simulink model "FeedbackLin"  (R2016a)
settings: Solver=ode45  StartTime=0.0  StopTime=2*Tpasso  FixedStep=1e-4  RelTol=1e-5
values from neighbouring files (symbols this model uses):
  Bm = 1e-4    (= 0.0001)    [runTests.m]
  cm = [c1; c2; c3; c4; c5]    [runTests.m]
  Cphi = 1    [runTests.m]
  cr = [c1; c2; c3; c4; c5]    [runTests.m]
  dQ0 = [dQ10; dQ20; dQ30; dQ40; dQ50]    [runNoErrorNoNoiseNoIncNoFext.m]    (also in runTests.m = zeros(5,1))
  gait = 1    [runTests.m]
  gm = g    (= 9.81)    [runTests.m]
  gr = g    (= 9.81)    [runTests.m]
  Im = [I1; I2; I3; I4; I5]    [runTests.m]
  Ir = [I1; I2; I3; I4; I5]    [runTests.m]
  Jm = 5e-3    (= 0.005)    [runTests.m]
  Kt = 0.1    [runTests.m]
  La = 1e-3    (= 0.001)    [runTests.m]
  LambdaFL = [150; 150; 150; 150]    [runTests.m]
  lm = [l1; l2; l3; l4; l5]    [runTests.m]
  lr = [l1; l2; l3; l4; l5]    [runTests.m]
  mInc = tan(Inc*pi/180)    [runTests.m]
  mm = [m1; m2; m3; m4; m5]    [runTests.m]
  mr = [m1; m2; m3; m4; m5]    [runTests.m]
  pertAmp = 0    [runTests.m]
  pertDur = 0    [runTests.m]
  pertStep = 0    [runTests.m]
  Q0 = [Q10; Q20; Q30; Q40; Q50]    [runNoErrorNoNoiseNoIncNoFext.m]    (also in runTests.m = [pi/2 - pi/10; pi/5; 2*pi-pi/10; pi+pi/10; -pi/4.5])
  Ra = 1    [runTests.m]
  Tpasso = 0.35    [runTests.m]
  TsC = 0.003    [runTests.m]
  TsPID = 1/1000    (= 0.001)    [runTests.m]
  useNoise = false    [runTests.m]
undefined symbols (not defined in the file or in its folder): curStep, Rp1, Rp2
libraries: simulink x8, commrandsrc3 x2
(part 1 of 3)
settings Model: Creator=PPA  LastModifiedBy=Barth

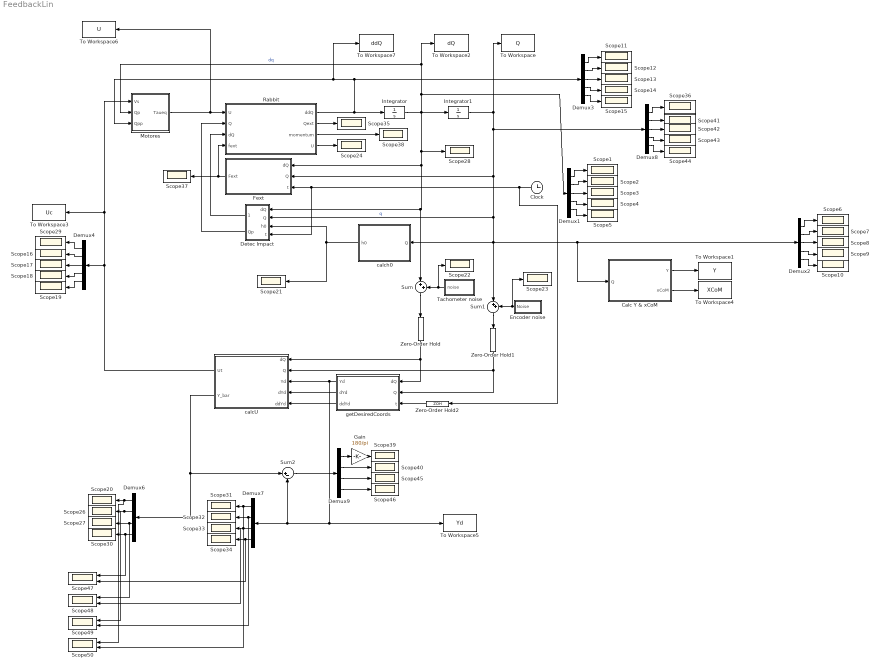
== system FeedbackLin ==
  Calc Y & xCoM : MATLAB Function  TreatAsAtomicUnit=on  SystemSampleTime=TsC
  Clock : Clock
  Demux{1..4,8} (5 alike) : Demux  Outputs=5
  Demux6 : Demux
  Demux7 : Demux
  Demux9 : Demux
  Detec Impact : Subsystem
  Encoder noise : Subsystem
  Fext : MATLAB Function  TreatAsAtomicUnit=on
  Gain : Gain  Gain=180/pi
  Integrator : Integrator  InitialCondition=dQ0
  Integrator1 : Integrator  InitialCondition=Q0
  Motores : Subsystem
  Rabbit : MATLAB Function  TreatAsAtomicUnit=on
  Scope{1..24,26..46} (45 alike) : Scope
  Scope{47..50} (4 alike) : Scope  NumInputPorts=2
  Sum : Sum  Inputs=|++
  Sum1 : Sum  Inputs=|++
  Sum2 : Sum  Inputs=|+-
  Tachometer noise : Subsystem
  To Workspace : ToWorkspace  VariableName=Q  SaveFormat=Structure With Time  SampleTime=-1
  To Workspace1 : ToWorkspace  VariableName=Y  SaveFormat=Structure With Time  SampleTime=-1
  To Workspace2 : ToWorkspace  VariableName=dQ  SaveFormat=Structure With Time  SampleTime=-1
  To Workspace3 : ToWorkspace  VariableName=Uc  SaveFormat=Structure With Time  SampleTime=-1
  To Workspace4 : ToWorkspace  VariableName=XCoM  SaveFormat=Structure With Time  SampleTime=-1
  To Workspace5 : ToWorkspace  VariableName=Yd  SaveFormat=Structure With Time  SampleTime=-1
  To Workspace6 : ToWorkspace  VariableName=U  SaveFormat=Structure With Time  SampleTime=-1
  To Workspace7 : ToWorkspace  VariableName=ddQ  SaveFormat=Structure With Time  SampleTime=-1
  Zero-Order Hold : ZeroOrderHold  SampleTime=TsC
  Zero-Order Hold1 : ZeroOrderHold  SampleTime=TsC
  Zero-Order Hold2 : ZeroOrderHold  SampleTime=TsC
  calcU : MATLAB Function  TreatAsAtomicUnit=on  SystemSampleTime=TsC
  calch0 : MATLAB Function  TreatAsAtomicUnit=on
  getDesiredCoords : Subsystem
  wires:
  Demux3/1 -> Scope11/1
  Demux3/2 -> Scope12/1
  Demux3/3 -> Scope13/1
  Demux3/4 -> Scope14/1
  Demux3/5 -> Scope15/1
  Integrator/1 -> Motores/2(Qp), To Workspace2/1, Demux1/1, Fext/1(dQ), Detec Impact/1(dQ), Sum/1, Scope28/1, Integrator1/1  "dq"
  Integrator1/1 -> Fext/2(Q), Detec Impact/2(Q), Calc Y & xCoM/1(Q), Demux2/1, Sum1/1, calch0/1(Q), Demux8/1, To Workspace/1  "q"
  Demux1/1 -> Scope1/1
  Demux1/2 -> Scope2/1
  Demux1/3 -> Scope3/1
  Demux1/4 -> Scope4/1
  Demux1/5 -> Scope5/1
  Demux2/1 -> Scope6/1
  Demux2/2 -> Scope7/1
  Demux2/3 -> Scope8/1
  Demux2/4 -> Scope9/1
  Demux2/5 -> Scope10/1
  Fext/1(Fext) -> Rabbit/4(fext), Scope37/1
  Clock/1 -> Zero-Order Hold2/1, Fext/3(t), Detec Impact/4(t)
  Demux4/3 -> Scope17/1
  Demux4/2 -> Scope16/1
  Demux4/1 -> Scope29/1
  Demux4/4 -> Scope18/1
  Demux4/5 -> Scope19/1
  Sum/1 -> Zero-Order Hold/1
  Sum1/1 -> Zero-Order Hold1/1
  Rabbit/3(momentum) -> Scope38/1
  Tachometer noise/1(noise) -> Sum/2, Scope22/1
  Detec Impact/1(dQp) -> Rabbit/3(dQ)
  Detec Impact/2(Qp) -> Rabbit/2(Q)
  calch0/1(h0) -> Scope21/1, Detec Impact/3(h0)
  Rabbit/2(Qext) -> Scope35/1
  Rabbit/1(ddQ) -> Demux3/1, To Workspace7/1, Motores/3(Qpp), Integrator/1
  Demux8/1 -> Scope36/1
  Demux8/2 -> Scope41/1
  Demux8/3 -> Scope42/1
  Demux8/4 -> Scope43/1
  Demux8/5 -> Scope44/1
  getDesiredCoords/3(ddYd) -> calcU/5(ddYd)
  getDesiredCoords/2(dYd) -> calcU/4(dYd)
  getDesiredCoords/1(Yd) -> calcU/3(Yd), To Workspace5/1, Sum2/2, Demux7/1
  Demux6/3 -> Scope48/1, Scope27/1
  Demux6/2 -> Scope49/1, Scope26/1
  Demux6/1 -> Scope50/1, Scope20/1
  Demux6/4 -> Scope47/1, Scope30/1
  Demux7/3 -> Scope48/2, Scope33/1
  Demux7/2 -> Scope49/2, Scope32/1
  Demux7/1 -> Scope50/2, Scope31/1
  Demux7/4 -> Scope47/2, Scope34/1
  Demux9/3 -> Scope45/1
  Demux9/2 -> Scope40/1
  Demux9/1 -> Gain/1
  Demux9/4 -> Scope46/1
  Sum2/1 -> Demux9/1
  Gain/1 -> Scope39/1
  Motores/1(Taueq) -> To Workspace6/1, Rabbit/1("U ")
  calcU/2(Y_bar) -> Demux6/1, Sum2/1
  calcU/1(Ut) -> Motores/1(Vs), To Workspace3/1, Demux4/1
  Zero-Order Hold/1 -> calcU/1(dQ), getDesiredCoords/1(dQ)
  Zero-Order Hold1/1 -> calcU/2(Q), getDesiredCoords/2(Q)
  Zero-Order Hold2/1 -> getDesiredCoords/3(t)
  Calc Y & xCoM/2(xCoM) -> To Workspace4/1
  Calc Y & xCoM/1(Y) -> To Workspace1/1
  Encoder noise/1(Noise) -> Sum1/2, Scope23/1
  Rabbit/4(U) -> Scope24/1

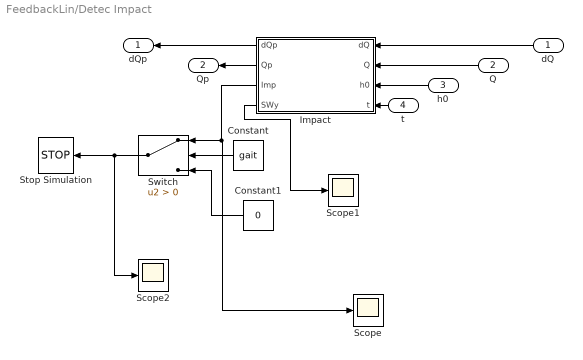
== system FeedbackLin/Detec Impact ==
  dQ : Inport
  Q : Inport  Port=2
  h0 : Inport  Port=3
  t : Inport  Port=4
  Constant : Constant  Value=gait
  Constant1 : Constant  Value=0
  Impact : MATLAB Function  TreatAsAtomicUnit=on
  Scope : Scope
  Scope1 : Scope
  Scope2 : Scope
  Stop Simulation : Stop
  Switch : Switch  Criteria=u2 > Threshold
  dQp : Outport
  Qp : Outport  Port=2
  wires:
  Impact/2(Qp) -> Qp/1
  Impact/1(dQp) -> dQp/1
  Impact/3(Imp) -> Switch/1, Scope/1
  dQ/1 -> Impact/1(dQ)
  Constant1/1 -> Switch/3
  Constant/1 -> Switch/2
  h0/1 -> Impact/3(h0)
  Q/1 -> Impact/2(Q)
  t/1 -> Impact/4(t)
  Impact/4(SWy) -> Scope1/1
  Switch/1 -> Stop Simulation/1, Scope2/1

== system FeedbackLin/Encoder noise ==
  Constant : Constant  Value=useNoise
  Constant1 : Constant  Value=0
  Gain : Gain  Gain=0.002
  Scope27 : Scope
  Subsystem2 : Subsystem
  Switch : Switch  Criteria=u2 > Threshold
  Noise : Outport
  wires:
  Subsystem2/1("Bernouli ") -> Gain/1
  Constant/1 -> Switch/2
  Gain/1 -> Switch/1, Scope27/1
  Switch/1 -> Noise/1
  Constant1/1 -> Switch/3

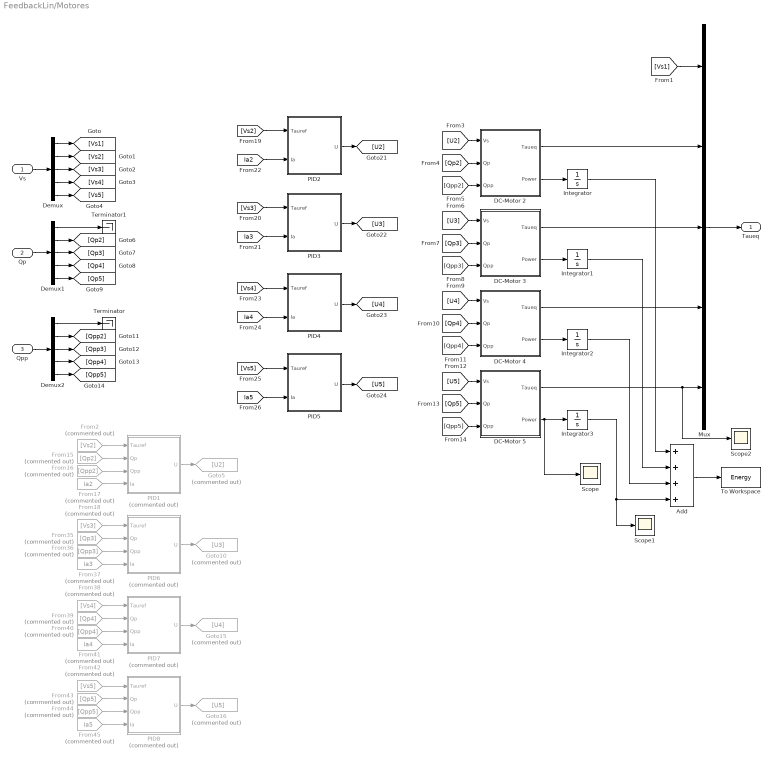
== system FeedbackLin/Motores ==
  Vs : Inport
  Qp : Inport  Port=2
  Qpp : Inport  Port=3
  Add : Sum  Inputs=++++
  DC-Motor 2 : Subsystem
  DC-Motor 3 : Subsystem
  DC-Motor 4 : Subsystem
  DC-Motor 5 : Subsystem
  Demux : Demux  Outputs=5
  Demux1 : Demux  Outputs=5
  Demux2 : Demux  Outputs=5
  From15 : From  Commented=on  GotoTag=Qp2
  From16 : From  Commented=on  GotoTag=Qpp2
  From17 : From  Commented=on  GotoTag=Ia2  TagVisibility=global
  From18 : From  Commented=on  GotoTag=Vs3
  From2 : From  Commented=on  GotoTag=Vs2
  From35 : From  Commented=on  GotoTag=Qp3
  From36 : From  Commented=on  GotoTag=Qpp3
  From37 : From  Commented=on  GotoTag=Ia3  TagVisibility=global
  From38 : From  Commented=on  GotoTag=Vs4
  From39 : From  Commented=on  GotoTag=Qp4
  From40 : From  Commented=on  GotoTag=Qpp4
  From41 : From  Commented=on  GotoTag=Ia4  TagVisibility=global
  From42 : From  Commented=on  GotoTag=Vs5
  From43 : From  Commented=on  GotoTag=Qp5
  From44 : From  Commented=on  GotoTag=Qpp5
  From45 : From  Commented=on  GotoTag=Ia5  TagVisibility=global
  Goto10 : Goto  Commented=on  GotoTag=U3
  Goto15 : Goto  Commented=on  GotoTag=U4
  Goto16 : Goto  Commented=on  GotoTag=U5
  Goto5 : Goto  Commented=on  GotoTag=U2
  Integrator{,1..3} (4 alike) : Integrator
  Mux : Mux  Inputs=5
  PID1 : Subsystem  Commented=on
  PID2 : Subsystem
  PID3 : Subsystem
  PID4 : Subsystem
  PID5 : Subsystem
  PID6 : Subsystem  Commented=on
  PID7 : Subsystem  Commented=on
  PID8 : Subsystem  Commented=on
  Scope : Scope
  Scope1 : Scope
  Scope2 : Scope
  Terminator : Terminator
  Terminator1 : Terminator
  To Workspace : ToWorkspace  VariableName=Energy  SaveFormat=Structure With Time  SampleTime=-1
  Taueq : Outport  PortDimensions=5
  wires:
  [Vs1] -> Mux/1
  Vs/1 -> Demux/1
  Qp/1 -> Demux1/1
  Qpp/1 -> Demux2/1
  Demux/1 -> [Vs1]
  Demux/2 -> [Vs2]
  Demux/3 -> [Vs3]
  Demux/4 -> [Vs4]
  Demux/5 -> [Vs5]
  Demux1/1 -> Terminator1/1
  Demux1/2 -> [Qp2]
  Demux1/3 -> [Qp3]
  Demux1/4 -> [Qp4]
  Demux1/5 -> [Qp5]
  Demux2/1 -> Terminator/1
  Demux2/2 -> [Qpp2]
  Demux2/3 -> [Qpp3]
  Demux2/4 -> [Qpp4]
  Demux2/5 -> [Qpp5]
  [U2] -> DC-Motor 2/1(Vs)
  [Qp2] -> DC-Motor 2/2(Qp)
  [Qpp2] -> DC-Motor 2/3(Qpp)
  [U3] -> DC-Motor 3/1(Vs)
  [Qp3] -> DC-Motor 3/2(Qp)
  [Qpp3] -> DC-Motor 3/3(Qpp)
  [U4] -> DC-Motor 4/1(Vs)
  [Qp4] -> DC-Motor 4/2(Qp)
  [Qpp4] -> DC-Motor 4/3(Qpp)
  [U5] -> DC-Motor 5/1(Vs)
  [Qp5] -> DC-Motor 5/2(Qp)
  [Qpp5] -> DC-Motor 5/3(Qpp)
  Mux/1 -> Taueq/1
  DC-Motor 2/1(Taueq) -> Mux/2
  DC-Motor 4/1(Taueq) -> Mux/4
  DC-Motor 3/1(Taueq) -> Mux/3
  DC-Motor 5/1(Taueq) -> Mux/5, Scope2/1
  PID2/1(U) -> [U2]
  PID3/1(U) -> [U3]
  PID4/1(U) -> [U4]
  PID5/1(U) -> [U5]
  [Ia2] -> PID2/2(Ia)
  [Vs2] -> PID2/1(Tauref)
  PID1/1(U) -> Goto5/1
  PID6/1(U) -> Goto10/1
  PID7/1(U) -> Goto15/1
  PID8/1(U) -> Goto16/1
  From42/1 -> PID8/1(Tauref)
  From43/1 -> PID8/2(Qp)
  From44/1 -> PID8/3(Qpp)
  From45/1 -> PID8/4(Ia)
  From41/1 -> PID7/4(Ia)
  From40/1 -> PID7/3(Qpp)
  From39/1 -> PID7/2(Qp)
  From38/1 -> PID7/1(Tauref)
  From37/1 -> PID6/4(Ia)
  From36/1 -> PID6/3(Qpp)
  From35/1 -> PID6/2(Qp)
  From18/1 -> PID6/1(Tauref)
  From17/1 -> PID1/4(Ia)
  From16/1 -> PID1/3(Qpp)
  From15/1 -> PID1/2(Qp)
  From2/1 -> PID1/1(Tauref)
  [Ia3] -> PID3/2(Ia)
  [Vs3] -> PID3/1(Tauref)
  [Ia4] -> PID4/2(Ia)
  [Vs4] -> PID4/1(Tauref)
  [Ia5] -> PID5/2(Ia)
  [Vs5] -> PID5/1(Tauref)
  DC-Motor 2/2(Power) -> Integrator/1
  DC-Motor 4/2(Power) -> Integrator2/1
  DC-Motor 3/2(Power) -> Integrator1/1
  Integrator3/1 -> Scope1/1, Add/4
  Integrator2/1 -> Add/3
  Integrator1/1 -> Add/2
  Integrator/1 -> Add/1
  Add/1 -> To Workspace/1
  DC-Motor 5/2(Power) -> Scope/1, Integrator3/1

== system FeedbackLin/Tachometer noise ==
  Constant : Constant  Value=useNoise
  Constant1 : Constant  Value=0
  Random Number : RandomNumber  Variance=10e-7  Seed=17  SampleTime=TsC
  Scope39 : Scope
  Switch : Switch  Criteria=u2 > Threshold
  noise : Outport
  wires:
  Constant/1 -> Switch/2
  Switch/1 -> noise/1
  Random Number/1 -> Switch/1, Scope39/1
  Constant1/1 -> Switch/3

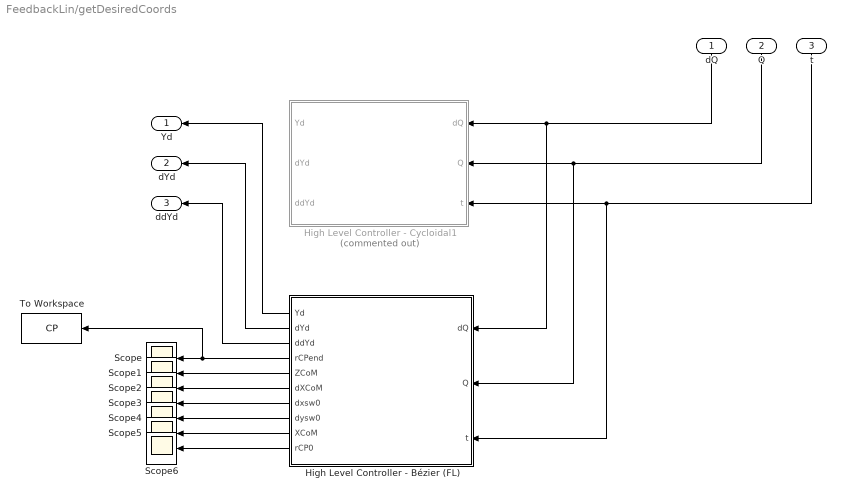
== system FeedbackLin/getDesiredCoords ==
  dQ : Inport
  Q : Inport  Port=2
  t : Inport  Port=3
  High Level Controller - Bézier (FL) : MATLAB Function  TreatAsAtomicUnit=on  SystemSampleTime=TsC
  High Level Controller - Cycloidal1 : MATLAB Function  Commented=on  TreatAsAtomicUnit=on
  Scope{,1..6} (7 alike) : Scope
  To Workspace : ToWorkspace  VariableName=CP  SaveFormat=Structure With Time  SampleTime=-1
  Yd : Outport
  dYd : Outport  Port=2
  ddYd : Outport  Port=3
  wires:
  t/1 -> High Level Controller - Bézier (FL)/3(t), High Level Controller - Cycloidal1/3(t)
  dQ/1 -> High Level Controller - Bézier (FL)/1(dQ), High Level Controller - Cycloidal1/1(dQ)
  Q/1 -> High Level Controller - Bézier (FL)/2(Q), High Level Controller - Cycloidal1/2(Q)
  High Level Controller - Bézier (FL)/1(Yd) -> Yd/1
  High Level Controller - Bézier (FL)/2(dYd) -> dYd/1
  High Level Controller - Bézier (FL)/3(ddYd) -> ddYd/1
  High Level Controller - Bézier (FL)/6(dXCoM) -> Scope2/1
  High Level Controller - Bézier (FL)/4(rCPend) -> To Workspace/1, Scope/1
  High Level Controller - Bézier (FL)/5(ZCoM) -> Scope1/1
  High Level Controller - Bézier (FL)/7(dxsw0) -> Scope3/1
  High Level Controller - Bézier (FL)/8(dysw0) -> Scope4/1
  High Level Controller - Bézier (FL)/9(XCoM) -> Scope5/1
  High Level Controller - Bézier (FL)/10(rCP0) -> Scope6/1

== system FeedbackLin/Encoder noise/Subsystem2 ==
  Bernoulli Binary Generator : commrandsrc3/Bernoulli Binary Generator  ProbabilityOfZero=0.99  SeedSource=Parameter  Seed=9745  SampleTime=TsC  SamplesPerFrame=1  OutputDataType=double  SimulateUsing=Interpreted execution
  Bernoulli Binary Generator1 : commrandsrc3/Bernoulli Binary Generator  ProbabilityOfZero=0.99  SeedSource=Parameter  Seed=8849  SampleTime=TsC  SamplesPerFrame=1  OutputDataType=double  SimulateUsing=Interpreted execution
  Sum2 : Sum  Inputs=|+-
  "Bernouli " : Outport
  wires:
  Sum2/1 -> "Bernouli "/1
  Bernoulli Binary Generator1/1 -> Sum2/2
  Bernoulli Binary Generator/1 -> Sum2/1

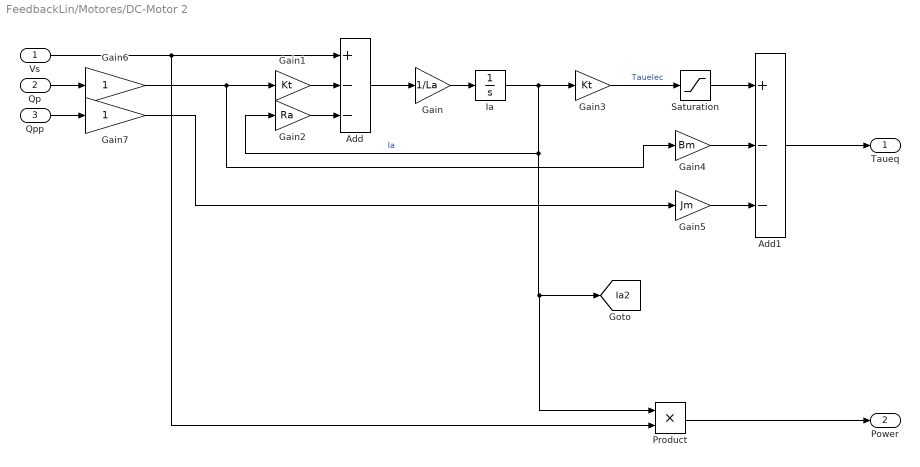
== system FeedbackLin/Motores/DC-Motor 2 ==
  Vs : Inport
  Qp : Inport  Port=2
  Qpp : Inport  Port=3
  Add : Sum  Inputs=+--
  Add1 : Sum  Inputs=+--
  Gain : Gain  Gain=1/La
  Gain1 : Gain  Gain=Kt
  Gain2 : Gain  Gain=Ra
  Gain3 : Gain  Gain=Kt
  Gain4 : Gain  Gain=Bm
  Gain5 : Gain  Gain=Jm
  Gain6 : Gain
  Gain7 : Gain
  Ia : Integrator
  Product : Product
  Saturation : Saturate  UpperLimit=inf  LowerLimit=-inf
  Taueq : Outport
  Power : Outport  Port=2
  tag scope: Ia2=global
  wires:
  Gain7/1 -> Gain5/1
  Gain6/1 -> Gain1/1, Gain4/1
  Qpp/1 -> Gain7/1
  Qp/1 -> Gain6/1
  Add/1 -> Gain/1
  Ia/1 -> Product/1, [Ia2], Gain2/1, Gain3/1  "Ia"
  Gain3/1 -> Saturation/1  "Tauelec"
  Gain/1 -> Ia/1
  Vs/1 -> Add/1, Product/2
  Gain4/1 -> Add1/2
  Gain5/1 -> Add1/3
  Gain2/1 -> Add/3
  Gain1/1 -> Add/2
  Add1/1 -> Taueq/1
  Saturation/1 -> Add1/1
  Product/1 -> Power/1

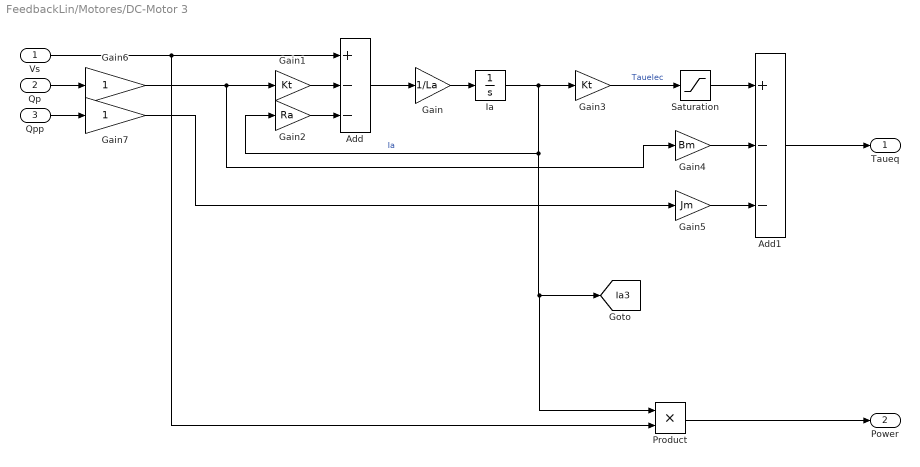
== system FeedbackLin/Motores/DC-Motor 3 ==
  Vs : Inport
  Qp : Inport  Port=2
  Qpp : Inport  Port=3
  Add : Sum  Inputs=+--
  Add1 : Sum  Inputs=+--
  Gain : Gain  Gain=1/La
  Gain1 : Gain  Gain=Kt
  Gain2 : Gain  Gain=Ra
  Gain3 : Gain  Gain=Kt
  Gain4 : Gain  Gain=Bm
  Gain5 : Gain  Gain=Jm
  Gain6 : Gain
  Gain7 : Gain
  Ia : Integrator
  Product : Product
  Saturation : Saturate  UpperLimit=inf  LowerLimit=-inf
  Taueq : Outport
  Power : Outport  Port=2
  tag scope: Ia3=global
  wires:
  Product/1 -> Power/1
  Saturation/1 -> Add1/1
  Add1/1 -> Taueq/1
  Gain1/1 -> Add/2
  Gain2/1 -> Add/3
  Gain5/1 -> Add1/3
  Gain4/1 -> Add1/2
  Vs/1 -> Product/2, Add/1
  Gain/1 -> Ia/1
  Gain3/1 -> Saturation/1  "Tauelec"
  Ia/1 -> Gain3/1, Gain2/1, [Ia3], Product/1  "Ia"
  Add/1 -> Gain/1
  Qp/1 -> Gain6/1
  Qpp/1 -> Gain7/1
  Gain6/1 -> Gain4/1, Gain1/1
  Gain7/1 -> Gain5/1

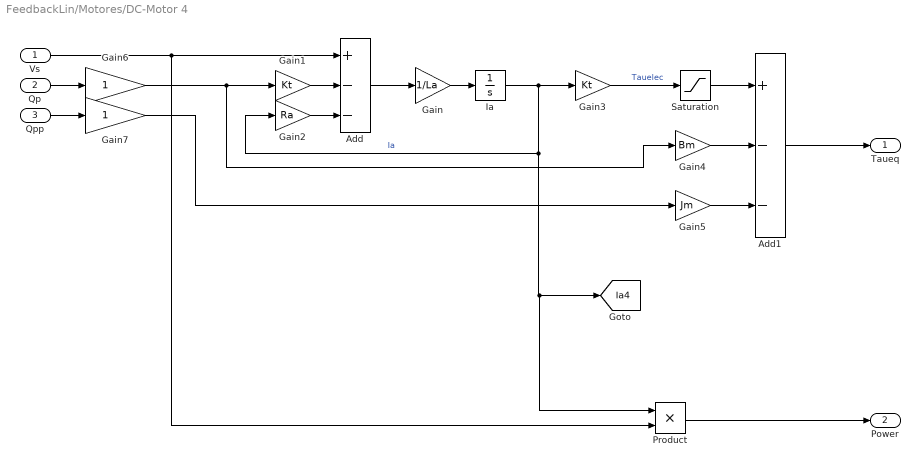
== system FeedbackLin/Motores/DC-Motor 4 ==
  Vs : Inport
  Qp : Inport  Port=2
  Qpp : Inport  Port=3
  Add : Sum  Inputs=+--
  Add1 : Sum  Inputs=+--
  Gain : Gain  Gain=1/La
  Gain1 : Gain  Gain=Kt
  Gain2 : Gain  Gain=Ra
  Gain3 : Gain  Gain=Kt
  Gain4 : Gain  Gain=Bm
  Gain5 : Gain  Gain=Jm
  Gain6 : Gain
  Gain7 : Gain
  Ia : Integrator
  Product : Product
  Saturation : Saturate  UpperLimit=inf  LowerLimit=-inf
  Taueq : Outport
  Power : Outport  Port=2
  tag scope: Ia4=global
  wires:
  Gain7/1 -> Gain5/1
  Gain6/1 -> Gain1/1, Gain4/1
  Qpp/1 -> Gain7/1
  Qp/1 -> Gain6/1
  Add/1 -> Gain/1
  Ia/1 -> Product/1, [Ia4], Gain2/1, Gain3/1  "Ia"
  Gain3/1 -> Saturation/1  "Tauelec"
  Gain/1 -> Ia/1
  Vs/1 -> Add/1, Product/2
  Gain4/1 -> Add1/2
  Gain5/1 -> Add1/3
  Gain2/1 -> Add/3
  Gain1/1 -> Add/2
  Add1/1 -> Taueq/1
  Saturation/1 -> Add1/1
  Product/1 -> Power/1

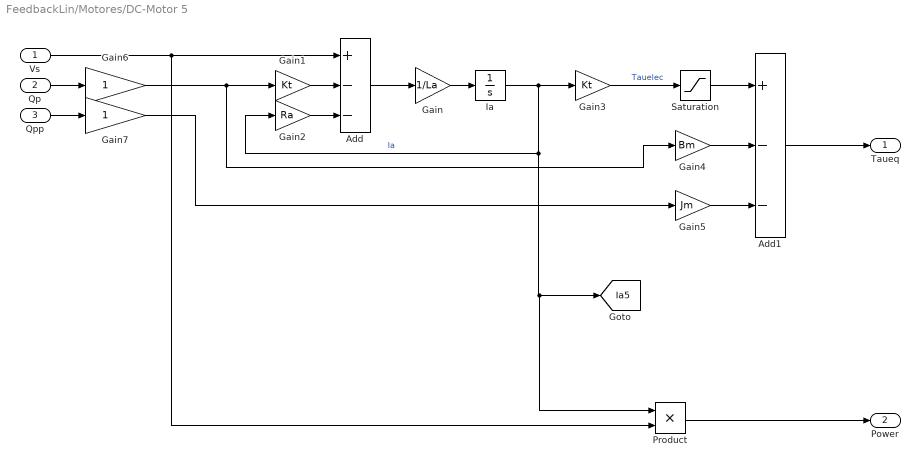
== system FeedbackLin/Motores/DC-Motor 5 ==
  Vs : Inport
  Qp : Inport  Port=2
  Qpp : Inport  Port=3
  Add : Sum  Inputs=+--
  Add1 : Sum  Inputs=+--
  Gain : Gain  Gain=1/La
  Gain1 : Gain  Gain=Kt
  Gain2 : Gain  Gain=Ra
  Gain3 : Gain  Gain=Kt
  Gain4 : Gain  Gain=Bm
  Gain5 : Gain  Gain=Jm
  Gain6 : Gain
  Gain7 : Gain
  Ia : Integrator
  Product : Product
  Saturation : Saturate  UpperLimit=inf  LowerLimit=-inf
  Taueq : Outport
  Power : Outport  Port=2
  tag scope: Ia5=global
  wires:
  Product/1 -> Power/1
  Saturation/1 -> Add1/1
  Add1/1 -> Taueq/1
  Gain1/1 -> Add/2
  Gain2/1 -> Add/3
  Gain5/1 -> Add1/3
  Gain4/1 -> Add1/2
  Vs/1 -> Product/2, Add/1
  Gain/1 -> Ia/1
  Gain3/1 -> Saturation/1  "Tauelec"
  Ia/1 -> Gain3/1, Gain2/1, [Ia5], Product/1  "Ia"
  Add/1 -> Gain/1
  Qp/1 -> Gain6/1
  Qpp/1 -> Gain7/1
  Gain6/1 -> Gain4/1, Gain1/1
  Gain7/1 -> Gain5/1

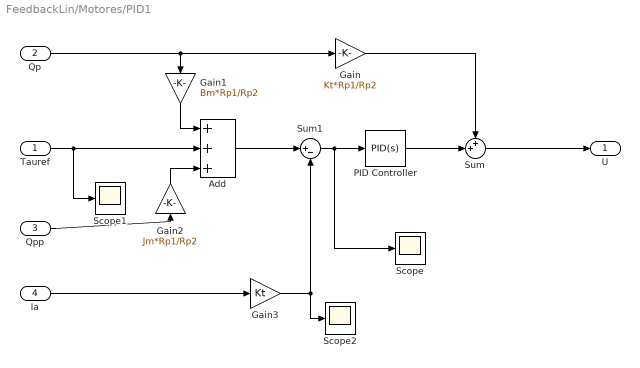
== system FeedbackLin/Motores/PID1 ==
  Tauref : Inport
  Qp : Inport  Port=2
  Qpp : Inport  Port=3
  Ia : Inport  Port=4
  Add : Sum  Inputs=+++
  Gain : Gain  Gain=Kt*Rp1/Rp2
  Gain1 : Gain  Gain=Bm*Rp1/Rp2
  Gain2 : Gain  Gain=Jm*Rp1/Rp2
  Gain3 : Gain  Gain=Kt
  PID Controller : simulink/Continuous/PID Controller  Controller=PID  TimeDomain=Continuous-time  SampleTime=-1  IntegratorMethod=Forward Euler  FilterMethod=Forward Euler  Form=Parallel  UseFilter=on  ControllerParametersSource=internal  P=13  I=13000  D=0  N=100  InitialConditionSource=internal  InitialConditionForIntegrator=0  InitialConditionForFilter=0  ExternalReset=none  LimitOutput=off  UpperSaturationLimit=inf  LowerSaturationLimit=-inf  LinearizeAsGain=on  AntiWindupMode=none  Kb=1  TrackingMode=off  Kt=1  PParamMin=[]  PParamMax=[]  IParamMin=[]  IParamMax=[]  DParamMin=[]  DParamMax=[]  NParamMin=[]  NParamMax=[]  KbParamMin=[]  KbParamMax=[]  KtParamMin=[]  KtParamMax=[]  POutMin=[]  POutMax=[]  IOutMin=[]  IOutMax=[]  DOutMin=[]  DOutMax=[]  NOutMin=[]  NOutMax=[]  KbOutMin=[]  KbOutMax=[]  KtOutMin=[]  KtOutMax=[]  IntegratorOutMin=[]  IntegratorOutMax=[]  FilterOutMin=[]  FilterOutMax=[]  SumOutMin=[]  SumOutMax=[]  SumI1OutMin=[]  SumI1OutMax=[]  SumI2OutMin=[]  SumI2OutMax=[]  SumI3OutMin=[]  SumI3OutMax=[]  SumDOutMin=[]  SumDOutMax=[]  SaturationOutMin=[]  SaturationOutMax=[]  IntegratorContinuousStateAttributes=''  IntegratorStateMustResolveToSignalObject=off  IntegratorRTWStateStorageClass=Auto  FilterContinuousStateAttributes=''  FilterStateMustResolveToSignalObject=off  FilterRTWStateStorageClass=Auto  DifferentiatorICPrevScaledInput=0  DifferentiatorOutMin=[]  DifferentiatorOutMax=[]
  Scope : Scope
  Scope1 : Scope
  Scope2 : Scope
  Sum : Sum  Inputs=++|
  Sum1 : Sum  Inputs=|+-
  U : Outport
  wires:
  Ia/1 -> Gain3/1
  Qpp/1 -> Gain2/1
  Tauref/1 -> Scope1/1, Add/2
  Qp/1 -> Gain/1, Gain1/1
  Gain3/1 -> Sum1/2, Scope2/1
  Add/1 -> Sum1/1
  Sum1/1 -> Scope/1, PID Controller/1
  Gain2/1 -> Add/3
  Gain1/1 -> Add/1
  Sum/1 -> U/1
  Gain/1 -> Sum/1
  PID Controller/1 -> Sum/2

== system FeedbackLin/Motores/PID2 ==
  Tauref : Inport
  Ia : Inport  Port=2
  Gain3 : Gain  Gain=Kt
  Hs : simulink/Continuous/PID Controller  Controller=PI  TimeDomain=Discrete-time  SampleTime=TsPID  IntegratorMethod=Forward Euler  FilterMethod=Trapezoidal  Form=Parallel  UseFilter=on  ControllerParametersSource=internal  P=15  I=9853  D=0  N=10000  InitialConditionSource=internal  InitialConditionForIntegrator=0  InitialConditionForFilter=0  ExternalReset=none  LimitOutput=off  UpperSaturationLimit=inf  LowerSaturationLimit=-inf  LinearizeAsGain=on  AntiWindupMode=none  Kb=1  TrackingMode=off  Kt=1  PParamMin=[]  PParamMax=[]  IParamMin=[]  IParamMax=[]  DParamMin=[]  DParamMax=[]  NParamMin=[]  NParamMax=[]  KbParamMin=[]  KbParamMax=[]  KtParamMin=[]  KtParamMax=[]  POutMin=[]  POutMax=[]  IOutMin=[]  IOutMax=[]  DOutMin=[]  DOutMax=[]  NOutMin=[]  NOutMax=[]  KbOutMin=[]  KbOutMax=[]  KtOutMin=[]  KtOutMax=[]  IntegratorOutMin=[]  IntegratorOutMax=[]  FilterOutMin=[]  FilterOutMax=[]  SumOutMin=[]  SumOutMax=[]  SumI1OutMin=[]  SumI1OutMax=[]  SumI2OutMin=[]  SumI2OutMax=[]  SumI3OutMin=[]  SumI3OutMax=[]  SumDOutMin=[]  SumDOutMax=[]  SaturationOutMin=[]  SaturationOutMax=[]  IntegratorContinuousStateAttributes=''  IntegratorStateMustResolveToSignalObject=off  IntegratorRTWStateStorageClass=Auto  FilterContinuousStateAttributes=''  FilterStateMustResolveToSignalObject=off  FilterRTWStateStorageClass=Auto  DifferentiatorICPrevScaledInput=0  DifferentiatorOutMin=[]  DifferentiatorOutMax=[]
  Scope : Scope
  Scope1 : Scope
  Sum1 : Sum  Inputs=|+-
  Zero-Order Hold : ZeroOrderHold  SampleTime=TsPID
  Zero-Order Hold1 : ZeroOrderHold  SampleTime=TsPID
  U : Outport
  wires:
  Ia/1 -> Zero-Order Hold1/1
  Gain3/1 -> Sum1/2
  Sum1/1 -> Hs/1, Scope/1
  Hs/1 -> U/1
  Tauref/1 -> Zero-Order Hold/1
  Zero-Order Hold/1 -> Sum1/1
  Zero-Order Hold1/1 -> Scope1/1, Gain3/1

== system FeedbackLin/Motores/PID3 ==
  Tauref : Inport
  Ia : Inport  Port=2
  Gain3 : Gain  Gain=Kt
  Hs : simulink/Continuous/PID Controller  Controller=PI  TimeDomain=Discrete-time  SampleTime=TsPID  IntegratorMethod=Forward Euler  FilterMethod=Trapezoidal  Form=Parallel  UseFilter=on  ControllerParametersSource=internal  P=15  I=9853  D=0  N=10000  InitialConditionSource=internal  InitialConditionForIntegrator=0  InitialConditionForFilter=0  ExternalReset=none  LimitOutput=off  UpperSaturationLimit=inf  LowerSaturationLimit=-inf  LinearizeAsGain=on  AntiWindupMode=none  Kb=1  TrackingMode=off  Kt=1  PParamMin=[]  PParamMax=[]  IParamMin=[]  IParamMax=[]  DParamMin=[]  DParamMax=[]  NParamMin=[]  NParamMax=[]  KbParamMin=[]  KbParamMax=[]  KtParamMin=[]  KtParamMax=[]  POutMin=[]  POutMax=[]  IOutMin=[]  IOutMax=[]  DOutMin=[]  DOutMax=[]  NOutMin=[]  NOutMax=[]  KbOutMin=[]  KbOutMax=[]  KtOutMin=[]  KtOutMax=[]  IntegratorOutMin=[]  IntegratorOutMax=[]  FilterOutMin=[]  FilterOutMax=[]  SumOutMin=[]  SumOutMax=[]  SumI1OutMin=[]  SumI1OutMax=[]  SumI2OutMin=[]  SumI2OutMax=[]  SumI3OutMin=[]  SumI3OutMax=[]  SumDOutMin=[]  SumDOutMax=[]  SaturationOutMin=[]  SaturationOutMax=[]  IntegratorContinuousStateAttributes=''  IntegratorStateMustResolveToSignalObject=off  IntegratorRTWStateStorageClass=Auto  FilterContinuousStateAttributes=''  FilterStateMustResolveToSignalObject=off  FilterRTWStateStorageClass=Auto  DifferentiatorICPrevScaledInput=0  DifferentiatorOutMin=[]  DifferentiatorOutMax=[]
  Scope : Scope
  Scope1 : Scope
  Sum1 : Sum  Inputs=|+-
  Zero-Order Hold : ZeroOrderHold  SampleTime=TsPID
  Zero-Order Hold1 : ZeroOrderHold  SampleTime=TsPID
  U : Outport
  wires:
  Zero-Order Hold1/1 -> Gain3/1, Scope1/1
  Zero-Order Hold/1 -> Sum1/1
  Tauref/1 -> Zero-Order Hold/1
  Hs/1 -> U/1
  Sum1/1 -> Scope/1, Hs/1
  Gain3/1 -> Sum1/2
  Ia/1 -> Zero-Order Hold1/1

== system FeedbackLin/Motores/PID4 ==
  Tauref : Inport
  Ia : Inport  Port=2
  Gain3 : Gain  Gain=Kt
  Hs : simulink/Continuous/PID Controller  Controller=PI  TimeDomain=Discrete-time  SampleTime=TsPID  IntegratorMethod=Forward Euler  FilterMethod=Trapezoidal  Form=Parallel  UseFilter=on  ControllerParametersSource=internal  P=15  I=9853  D=0  N=10000  InitialConditionSource=internal  InitialConditionForIntegrator=0  InitialConditionForFilter=0  ExternalReset=none  LimitOutput=off  UpperSaturationLimit=inf  LowerSaturationLimit=-inf  LinearizeAsGain=on  AntiWindupMode=none  Kb=1  TrackingMode=off  Kt=1  PParamMin=[]  PParamMax=[]  IParamMin=[]  IParamMax=[]  DParamMin=[]  DParamMax=[]  NParamMin=[]  NParamMax=[]  KbParamMin=[]  KbParamMax=[]  KtParamMin=[]  KtParamMax=[]  POutMin=[]  POutMax=[]  IOutMin=[]  IOutMax=[]  DOutMin=[]  DOutMax=[]  NOutMin=[]  NOutMax=[]  KbOutMin=[]  KbOutMax=[]  KtOutMin=[]  KtOutMax=[]  IntegratorOutMin=[]  IntegratorOutMax=[]  FilterOutMin=[]  FilterOutMax=[]  SumOutMin=[]  SumOutMax=[]  SumI1OutMin=[]  SumI1OutMax=[]  SumI2OutMin=[]  SumI2OutMax=[]  SumI3OutMin=[]  SumI3OutMax=[]  SumDOutMin=[]  SumDOutMax=[]  SaturationOutMin=[]  SaturationOutMax=[]  IntegratorContinuousStateAttributes=''  IntegratorStateMustResolveToSignalObject=off  IntegratorRTWStateStorageClass=Auto  FilterContinuousStateAttributes=''  FilterStateMustResolveToSignalObject=off  FilterRTWStateStorageClass=Auto  DifferentiatorICPrevScaledInput=0  DifferentiatorOutMin=[]  DifferentiatorOutMax=[]
  Scope : Scope
  Scope1 : Scope
  Sum1 : Sum  Inputs=|+-
  Zero-Order Hold : ZeroOrderHold  SampleTime=TsPID
  Zero-Order Hold1 : ZeroOrderHold  SampleTime=TsPID
  U : Outport
  wires:
  Ia/1 -> Zero-Order Hold1/1
  Gain3/1 -> Sum1/2
  Sum1/1 -> Hs/1, Scope/1
  Hs/1 -> U/1
  Tauref/1 -> Zero-Order Hold/1
  Zero-Order Hold/1 -> Sum1/1
  Zero-Order Hold1/1 -> Scope1/1, Gain3/1

== system FeedbackLin/Motores/PID5 ==
  Tauref : Inport
  Ia : Inport  Port=2
  Gain3 : Gain  Gain=Kt
  Hs : simulink/Continuous/PID Controller  Controller=PI  TimeDomain=Discrete-time  SampleTime=TsPID  IntegratorMethod=Forward Euler  FilterMethod=Trapezoidal  Form=Parallel  UseFilter=on  ControllerParametersSource=internal  P=15  I=9853  D=0  N=10000  InitialConditionSource=internal  InitialConditionForIntegrator=0  InitialConditionForFilter=0  ExternalReset=none  LimitOutput=off  UpperSaturationLimit=inf  LowerSaturationLimit=-inf  LinearizeAsGain=on  AntiWindupMode=none  Kb=1  TrackingMode=off  Kt=1  PParamMin=[]  PParamMax=[]  IParamMin=[]  IParamMax=[]  DParamMin=[]  DParamMax=[]  NParamMin=[]  NParamMax=[]  KbParamMin=[]  KbParamMax=[]  KtParamMin=[]  KtParamMax=[]  POutMin=[]  POutMax=[]  IOutMin=[]  IOutMax=[]  DOutMin=[]  DOutMax=[]  NOutMin=[]  NOutMax=[]  KbOutMin=[]  KbOutMax=[]  KtOutMin=[]  KtOutMax=[]  IntegratorOutMin=[]  IntegratorOutMax=[]  FilterOutMin=[]  FilterOutMax=[]  SumOutMin=[]  SumOutMax=[]  SumI1OutMin=[]  SumI1OutMax=[]  SumI2OutMin=[]  SumI2OutMax=[]  SumI3OutMin=[]  SumI3OutMax=[]  SumDOutMin=[]  SumDOutMax=[]  SaturationOutMin=[]  SaturationOutMax=[]  IntegratorContinuousStateAttributes=''  IntegratorStateMustResolveToSignalObject=off  IntegratorRTWStateStorageClass=Auto  FilterContinuousStateAttributes=''  FilterStateMustResolveToSignalObject=off  FilterRTWStateStorageClass=Auto  DifferentiatorICPrevScaledInput=0  DifferentiatorOutMin=[]  DifferentiatorOutMax=[]
  Scope : Scope
  Scope1 : Scope
  Sum1 : Sum  Inputs=|+-
  Zero-Order Hold : ZeroOrderHold  SampleTime=TsPID
  Zero-Order Hold1 : ZeroOrderHold  SampleTime=TsPID
  U : Outport
  wires:
  Zero-Order Hold1/1 -> Gain3/1, Scope1/1
  Zero-Order Hold/1 -> Sum1/1
  Tauref/1 -> Zero-Order Hold/1
  Hs/1 -> U/1
  Sum1/1 -> Scope/1, Hs/1
  Gain3/1 -> Sum1/2
  Ia/1 -> Zero-Order Hold1/1

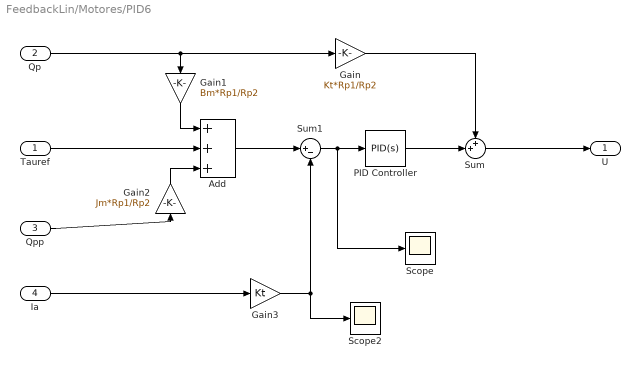
== system FeedbackLin/Motores/PID6 ==
  Tauref : Inport
  Qp : Inport  Port=2
  Qpp : Inport  Port=3
  Ia : Inport  Port=4
  Add : Sum  Inputs=+++
  Gain : Gain  Gain=Kt*Rp1/Rp2
  Gain1 : Gain  Gain=Bm*Rp1/Rp2
  Gain2 : Gain  Gain=Jm*Rp1/Rp2
  Gain3 : Gain  Gain=Kt
  PID Controller : simulink/Continuous/PID Controller  Controller=PID  TimeDomain=Continuous-time  SampleTime=-1  IntegratorMethod=Forward Euler  FilterMethod=Forward Euler  Form=Parallel  UseFilter=on  ControllerParametersSource=internal  P=13  I=13000  D=0  N=100  InitialConditionSource=internal  InitialConditionForIntegrator=0  InitialConditionForFilter=0  ExternalReset=none  LimitOutput=off  UpperSaturationLimit=inf  LowerSaturationLimit=-inf  LinearizeAsGain=on  AntiWindupMode=none  Kb=1  TrackingMode=off  Kt=1  PParamMin=[]  PParamMax=[]  IParamMin=[]  IParamMax=[]  DParamMin=[]  DParamMax=[]  NParamMin=[]  NParamMax=[]  KbParamMin=[]  KbParamMax=[]  KtParamMin=[]  KtParamMax=[]  POutMin=[]  POutMax=[]  IOutMin=[]  IOutMax=[]  DOutMin=[]  DOutMax=[]  NOutMin=[]  NOutMax=[]  KbOutMin=[]  KbOutMax=[]  KtOutMin=[]  KtOutMax=[]  IntegratorOutMin=[]  IntegratorOutMax=[]  FilterOutMin=[]  FilterOutMax=[]  SumOutMin=[]  SumOutMax=[]  SumI1OutMin=[]  SumI1OutMax=[]  SumI2OutMin=[]  SumI2OutMax=[]  SumI3OutMin=[]  SumI3OutMax=[]  SumDOutMin=[]  SumDOutMax=[]  SaturationOutMin=[]  SaturationOutMax=[]  IntegratorContinuousStateAttributes=''  IntegratorStateMustResolveToSignalObject=off  IntegratorRTWStateStorageClass=Auto  FilterContinuousStateAttributes=''  FilterStateMustResolveToSignalObject=off  FilterRTWStateStorageClass=Auto  DifferentiatorICPrevScaledInput=0  DifferentiatorOutMin=[]  DifferentiatorOutMax=[]
  Scope : Scope
  Scope2 : Scope
  Sum : Sum  Inputs=++|
  Sum1 : Sum  Inputs=|+-
  U : Outport
  wires:
  PID Controller/1 -> Sum/2
  Gain/1 -> Sum/1
  Sum/1 -> U/1
  Gain1/1 -> Add/1
  Gain2/1 -> Add/3
  Add/1 -> Sum1/1
  Qp/1 -> Gain1/1, Gain/1
  Tauref/1 -> Add/2
  Qpp/1 -> Gain2/1
  Ia/1 -> Gain3/1
  Gain3/1 -> Scope2/1, Sum1/2
  Sum1/1 -> PID Controller/1, Scope/1

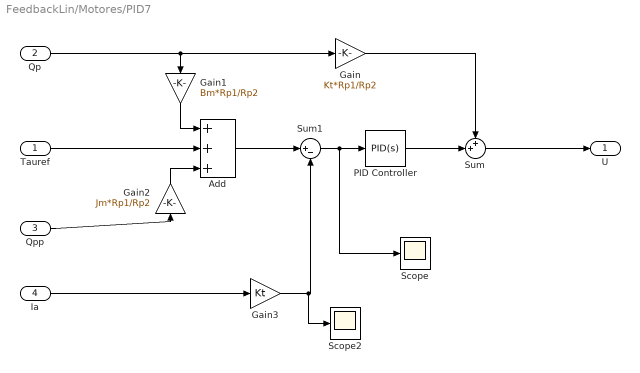
== system FeedbackLin/Motores/PID7 ==
  Tauref : Inport
  Qp : Inport  Port=2
  Qpp : Inport  Port=3
  Ia : Inport  Port=4
  Add : Sum  Inputs=+++
  Gain : Gain  Gain=Kt*Rp1/Rp2
  Gain1 : Gain  Gain=Bm*Rp1/Rp2
  Gain2 : Gain  Gain=Jm*Rp1/Rp2
  Gain3 : Gain  Gain=Kt
  PID Controller : simulink/Continuous/PID Controller  Controller=PID  TimeDomain=Continuous-time  SampleTime=-1  IntegratorMethod=Forward Euler  FilterMethod=Forward Euler  Form=Parallel  UseFilter=on  ControllerParametersSource=internal  P=13  I=13000  D=0  N=100  InitialConditionSource=internal  InitialConditionForIntegrator=0  InitialConditionForFilter=0  ExternalReset=none  LimitOutput=off  UpperSaturationLimit=inf  LowerSaturationLimit=-inf  LinearizeAsGain=on  AntiWindupMode=none  Kb=1  TrackingMode=off  Kt=1  PParamMin=[]  PParamMax=[]  IParamMin=[]  IParamMax=[]  DParamMin=[]  DParamMax=[]  NParamMin=[]  NParamMax=[]  KbParamMin=[]  KbParamMax=[]  KtParamMin=[]  KtParamMax=[]  POutMin=[]  POutMax=[]  IOutMin=[]  IOutMax=[]  DOutMin=[]  DOutMax=[]  NOutMin=[]  NOutMax=[]  KbOutMin=[]  KbOutMax=[]  KtOutMin=[]  KtOutMax=[]  IntegratorOutMin=[]  IntegratorOutMax=[]  FilterOutMin=[]  FilterOutMax=[]  SumOutMin=[]  SumOutMax=[]  SumI1OutMin=[]  SumI1OutMax=[]  SumI2OutMin=[]  SumI2OutMax=[]  SumI3OutMin=[]  SumI3OutMax=[]  SumDOutMin=[]  SumDOutMax=[]  SaturationOutMin=[]  SaturationOutMax=[]  IntegratorContinuousStateAttributes=''  IntegratorStateMustResolveToSignalObject=off  IntegratorRTWStateStorageClass=Auto  FilterContinuousStateAttributes=''  FilterStateMustResolveToSignalObject=off  FilterRTWStateStorageClass=Auto  DifferentiatorICPrevScaledInput=0  DifferentiatorOutMin=[]  DifferentiatorOutMax=[]
  Scope : Scope
  Scope2 : Scope
  Sum : Sum  Inputs=++|
  Sum1 : Sum  Inputs=|+-
  U : Outport
  wires:
  Ia/1 -> Gain3/1
  Qpp/1 -> Gain2/1
  Tauref/1 -> Add/2
  Qp/1 -> Gain/1, Gain1/1
  Add/1 -> Sum1/1
  Gain2/1 -> Add/3
  Gain1/1 -> Add/1
  Sum/1 -> U/1
  Gain/1 -> Sum/1
  PID Controller/1 -> Sum/2
  Gain3/1 -> Scope2/1, Sum1/2
  Sum1/1 -> Scope/1, PID Controller/1

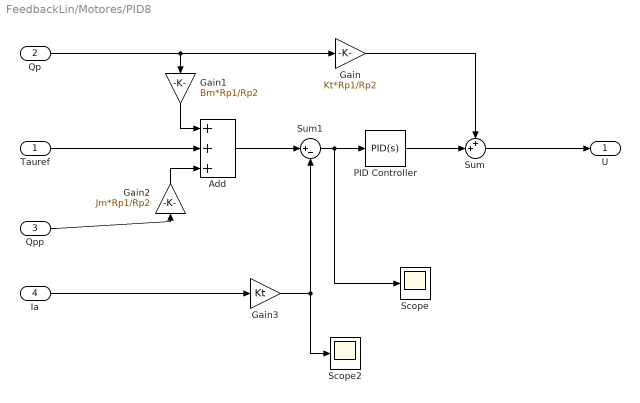
== system FeedbackLin/Motores/PID8 ==
  Tauref : Inport
  Qp : Inport  Port=2
  Qpp : Inport  Port=3
  Ia : Inport  Port=4
  Add : Sum  Inputs=+++
  Gain : Gain  Gain=Kt*Rp1/Rp2
  Gain1 : Gain  Gain=Bm*Rp1/Rp2
  Gain2 : Gain  Gain=Jm*Rp1/Rp2
  Gain3 : Gain  Gain=Kt
  PID Controller : simulink/Continuous/PID Controller  Controller=PID  TimeDomain=Continuous-time  SampleTime=-1  IntegratorMethod=Forward Euler  FilterMethod=Forward Euler  Form=Parallel  UseFilter=on  ControllerParametersSource=internal  P=13  I=13000  D=0  N=100  InitialConditionSource=internal  InitialConditionForIntegrator=0  InitialConditionForFilter=0  ExternalReset=none  LimitOutput=off  UpperSaturationLimit=inf  LowerSaturationLimit=-inf  LinearizeAsGain=on  AntiWindupMode=none  Kb=1  TrackingMode=off  Kt=1  PParamMin=[]  PParamMax=[]  IParamMin=[]  IParamMax=[]  DParamMin=[]  DParamMax=[]  NParamMin=[]  NParamMax=[]  KbParamMin=[]  KbParamMax=[]  KtParamMin=[]  KtParamMax=[]  POutMin=[]  POutMax=[]  IOutMin=[]  IOutMax=[]  DOutMin=[]  DOutMax=[]  NOutMin=[]  NOutMax=[]  KbOutMin=[]  KbOutMax=[]  KtOutMin=[]  KtOutMax=[]  IntegratorOutMin=[]  IntegratorOutMax=[]  FilterOutMin=[]  FilterOutMax=[]  SumOutMin=[]  SumOutMax=[]  SumI1OutMin=[]  SumI1OutMax=[]  SumI2OutMin=[]  SumI2OutMax=[]  SumI3OutMin=[]  SumI3OutMax=[]  SumDOutMin=[]  SumDOutMax=[]  SaturationOutMin=[]  SaturationOutMax=[]  IntegratorContinuousStateAttributes=''  IntegratorStateMustResolveToSignalObject=off  IntegratorRTWStateStorageClass=Auto  FilterContinuousStateAttributes=''  FilterStateMustResolveToSignalObject=off  FilterRTWStateStorageClass=Auto  DifferentiatorICPrevScaledInput=0  DifferentiatorOutMin=[]  DifferentiatorOutMax=[]
  Scope : Scope
  Scope2 : Scope
  Sum : Sum  Inputs=++|
  Sum1 : Sum  Inputs=|+-
  U : Outport
  wires:
  PID Controller/1 -> Sum/2
  Gain/1 -> Sum/1
  Sum/1 -> U/1
  Gain1/1 -> Add/1
  Gain2/1 -> Add/3
  Add/1 -> Sum1/1
  Qp/1 -> Gain1/1, Gain/1
  Tauref/1 -> Add/2
  Qpp/1 -> Gain2/1
  Ia/1 -> Gain3/1
  Gain3/1 -> Sum1/2, Scope2/1
  Sum1/1 -> Scope/1, PID Controller/1
